simulink model "Optical_Movement_Detection"  (Simulink 7.5)
settings: Solver=ode45  StartTime=0.0  StopTime=inf  RelTol=1e-3
values from neighbouring files (symbols this model uses):
  D = 1    [Copter_Animation.m]
  HSE_Bottom_1 = imresize(imread('D:\GoogleMapsBilder\PAR\HSE_Bottom_1.jpg'), 1)    [TESTS_Optical_Flow_Scenarios.m]
undefined symbols (not defined in the file or in its folder): dfilt, fspecial, imresize, Kanade, Low, Lucas, Rec, SDTV
libraries: simulink x17, dspobslib x12, vipgeotforms x5, dspsigops x4, dspmtrx3 x3, vipanalysis x3, dspstat3 x3, vipconversions x2, dspswit3 x2, vipsrcs x2, dsparch4 x1, dspsrcs4 x1
(part 1 of 2)
settings Model: Creator=roczit00  LastModifiedBy=Anonymos
settings DataIOCC: SaveOutput=off  DSMLogging=off  SaveTime=off
settings DebuggingCC: AlgebraicLoopMsg=none  SolverPrmCheckMsg=none  UnconnectedInputMsg=none  UnconnectedOutputMsg=none  UnconnectedLineMsg=none  StrictBusMsg=Warning

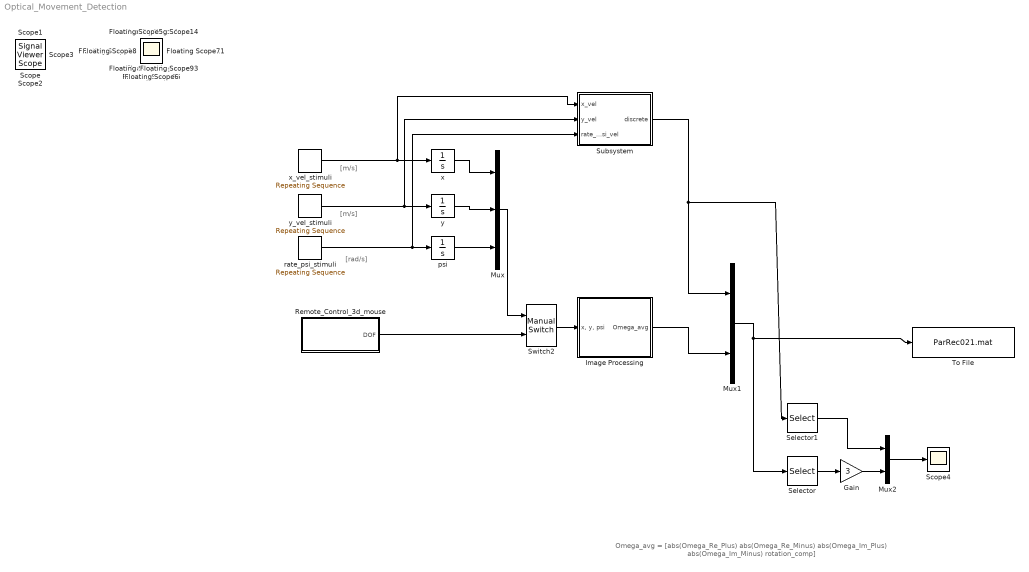
== system Optical_Movement_Detection ==
  note: [m/s]
  note: [m/s]
  note: [rad/s]
  note: Omega_avg = [abs(Omega_Re_Plus) abs(Omega_Re_Minus) abs(Omega_Im_Plus) abs(Omega_Im_Minus) rotation_comp]
  Gain : Gain  Gain=3  ParameterDataType=fixdt(1, 16)  ParameterScaling=2^0  OutDataType=fixdt(1, 16)  OutScaling=2^0
  Image Processing : Subsystem  mask{Ts_Opt=50, Cam_Img_Dim=[300,300], Env_Orig=[1300 1300], Block_Matching_Size=[31,31], Block_Matching_Overlap=[0 0], Block_Matching_Max_Disp=[7 7], Omega_avg_Gain=1/1000, load_cmd=HSE_Bottom_1}
      mask prompts: Ts_Opt "Camera's frames per second (1/SampleTime):"; Cam_Img_Dim "Cameras size of the synthetic image [R C]:"; Env_Orig "Initial image center of environment [R C]:"; Block_Matching_Size "Block size of optical flow block matching algorithm [heigh width]"; Block_Matching_Overlap "Block Overlap [R C] :"; Block_Matching_Max_Disp "Maximum displacement [R C]:"; Omega_avg_Gain "Gain of detected velocity vector"; load_cmd "Load Cmd"
      mask init:
      | set_param(gcb,'MaskSelfModifiable','on')
      mask TabNameString: General,General,General,Block Matching,Block Matching,Block Matching,Block Matching,General
  Mux : Mux  Inputs=3
  Mux1 : Mux  Inputs=2
  Mux2 : Mux  Inputs=2
  Remote_Control_3d_mouse : Subsystem  AncestorBlock=Remote_Control_Library/Remote_Control_3d_mouse
  Scope4 : Scope
      settings: TimeRange=1  YMin=0.25  YMax=4.5  SaveName=ScopeData9
  Selector : Selector  InputPortWidth=8  IndexOptions=Index vector (dialog)  Indices=[4]  OutputSizes=1
  Selector1 : Selector  InputPortWidth=3  IndexOptions=Index vector (dialog)  Indices=[1]  OutputSizes=1
  Subsystem : Subsystem  mask{In_Val_Sample_Time=0.01}
      mask prompts: In_Val_Sample_Time "Sample time"
  Switch2 : simulink/Signal Routing/Manual Switch  SystemSampleTime=-1  sw=1  action=0  varsize=off
  To File : ToFile  Filename=ParRec021.mat  MatrixName=Tfile
  psi : Integrator
  rate_psi_stimuli : simulink/Sources/Repeating Sequence  SystemSampleTime=-1  rep_seq_t=[0,5]  rep_seq_y=[0,-5]
  x : Integrator
  x_vel_stimuli : simulink/Sources/Repeating Sequence  SystemSampleTime=-1  rep_seq_t=[0,10]  rep_seq_y=[0,0]
  y : Integrator
  y_vel_stimuli : simulink/Sources/Repeating Sequence  SystemSampleTime=-1  rep_seq_t=[0,10]  rep_seq_y=[0,0]
  Floating Scope{,1..15} (16 alike) : Scope
      Floating Scope settings: Floating=on  YMin=-40  YMax=90
      Floating Scope1 settings: Floating=on
      Floating Scope10 settings: Floating=on  SaveName=ScopeData12
      Floating Scope11 settings: Floating=on  SaveName=ScopeData13
      Floating Scope12 settings: Floating=on  YMin=-2500  YMax=27500  SaveName=ScopeData14
      Floating Scope13 settings: Floating=on  YMin=3  YMax=7  SaveName=ScopeData15
      Floating Scope14 settings: Floating=on  SaveName=ScopeData16
      Floating Scope15 settings: Floating=on  SaveName=ScopeData17
      Floating Scope2 settings: Floating=on  YMin=-6000  YMax=2500  SaveName=ScopeData2
      Floating Scope3 settings: Floating=on  SaveName=ScopeData3
      Floating Scope4 settings: Floating=on  SaveName=ScopeData4
      Floating Scope5 settings: Floating=on  YMin=-0.7  YMax=0.8  SaveName=ScopeData5
      Floating Scope6 settings: Floating=on  YMin=-1  YMax=1  SaveName=ScopeData6
      Floating Scope7 settings: Floating=on  YMin=-15  YMax=10  SaveName=ScopeData7
      Floating Scope8 settings: Floating=on  YMax=45  SaveName=ScopeData10
      Floating Scope9 settings: Floating=on  YMin=-7  YMax=9  SaveName=ScopeData11
  Scope{,1..3} (4 alike) : SignalViewerScope  IOType=viewer  RefreshTime=0.035000
      Scope settings: YMin=-0.01  YMax=0.1
      Scope2 settings: SaveName=ScopeData2
      Scope3 settings: SaveName=ScopeData3
  wires:
  Remote_Control_3d_mouse/1(DOF) -> Switch2/2
  Mux/1 -> Switch2/1
  Switch2/1 -> Image Processing/1("x, y, psi")
  y_vel_stimuli/1 -> y/1, Subsystem/2(y_vel)
  x_vel_stimuli/1 -> x/1, Subsystem/1(x_vel)
  psi/1 -> Mux/3
  x/1 -> Mux/1
  y/1 -> Mux/2
  Mux1/1 -> Selector/1, To File/1
  Image Processing/1(Omega_avg) -> Mux1/2
  Mux2/1 -> Scope4/1
  Subsystem/1(discrete) -> Mux1/1, Selector1/1
  Selector/1 -> Gain/1
  Gain/1 -> Mux2/2
  Selector1/1 -> Mux2/1
  rate_psi_stimuli/1 -> psi/1, Subsystem/3(rate_psi_vel)

== system Optical_Movement_Detection/Image Processing ==
  note: Image Processing
  "x, y, psi" : Inport
  Allow Optical Flow : dspobslib/DSP Constant  SystemSampleTime=-1  Value=1  SampleMode=Discrete  discreteOutput=Sample-based  continuousOutput=Sample-based  sampTime=inf  framePeriod=2  dataType=boolean  isSigned=on  wordLen=16  udDataType=sfix(16)  fracBitsMode=Best precision  numFracBits=15  InterpretAs1D=-inf  Ts=-inf  FramebasedOutput=-inf
  Disable Optical Flow : dspobslib/DSP Constant  SystemSampleTime=-1  Value=0  SampleMode=Discrete  discreteOutput=Sample-based  continuousOutput=Sample-based  sampTime=inf  framePeriod=2  dataType=boolean  isSigned=on  wordLen=16  udDataType=sfix(16)  fracBitsMode=Best precision  numFracBits=15  InterpretAs1D=-inf  Ts=-inf  FramebasedOutput=-inf
  Input : Subsystem
      mask init:
      | set_param(gcb,'MaskSelfModifiable','on')
  Optical Flow : Subsystem
  Real Video : dspobslib/DSP Constant  SystemSampleTime=-1  Value=0  SampleMode=Discrete  discreteOutput=Sample-based  continuousOutput=Sample-based  sampTime=inf  framePeriod=2  dataType=boolean  isSigned=on  wordLen=16  udDataType=sfix(16)  fracBitsMode=Best precision  numFracBits=15  InterpretAs1D=-inf  Ts=-inf  FramebasedOutput=-inf
  Switch : simulink/Signal Routing/Manual Switch  SystemSampleTime=-1  sw=0  action=0  varsize=off
  Switch1 : simulink/Signal Routing/Manual Switch  SystemSampleTime=-1  sw=1  action=0  varsize=off
  Synthetic Video : dspobslib/DSP Constant  SystemSampleTime=-1  Value=1  SampleMode=Discrete  discreteOutput=Sample-based  continuousOutput=Sample-based  sampTime=inf  framePeriod=2  dataType=boolean  isSigned=on  wordLen=16  udDataType=sfix(16)  fracBitsMode=Best precision  numFracBits=15  InterpretAs1D=-inf  Ts=-inf  FramebasedOutput=-inf
  Omega_avg : Outport
  wires:
  Real Video/1 -> Switch/1
  Synthetic Video/1 -> Switch/2
  Switch/1 -> Input/1(Mode)
  "x, y, psi"/1 -> Input/2("x, y, psi")
  Input/1(Image) -> Optical Flow/1(Image)
  Input/2(I) -> Optical Flow/2(I)
  Allow Optical Flow/1 -> Switch1/1
  Disable Optical Flow/1 -> Switch1/2
  Optical Flow/1(Omega_avg) -> Omega_avg/1
  Switch1/1 -> Optical Flow/Enable

== system Optical_Movement_Detection/Remote_Control_3d_mouse ==
  Demux : Demux  Outputs=3
  Demux1 : Demux  Outputs=3
  Mux2 : Mux  Inputs=3
  Saturation : Saturate  UpperLimit=255  LowerLimit=-255
  Saturation1 : Saturate  UpperLimit=10  LowerLimit=-10
  Saturation2 : Saturate  UpperLimit=10  LowerLimit=-10
  Space Mouse Input : S-Function  AncestorBlock=vrlib/Space Mouse Input  FunctionName=spacemouse  Parameters=Port, OutputType, InitialPosition, InitialRotation, PositionSensitivity, RotationSensitivity, Dominant, NormalizeAngle, DisableTranslation, DisableRotation, PositionLow, PositionUp, EnableLimit  EnableBusSupport=off  mask(Space Mouse Input){Port=USB1, OutputType=Speed, Dominant=off, DisableTranslation=off, DisableRotation=off, NormalizeAngle=off, EnableLimit=on, PositionSensitivity=0.001, RotationSensitivity=0.001, InitialPosition=[0 0 0], InitialRotation=[0 0 0], PositionLow=[0 0 0], PositionUp=[255 255 255]}
      mask prompts: OutputType "Output type:"; Dominant "Dominant mode"; DisableTranslation "Disable position movement"; DisableRotation "Disable rotation movement"; NormalizeAngle "Normalize output angle"; EnableLimit "Limit position"; PositionSensitivity "Position sensitivity:"; RotationSensitivity "Rotation sensitivity:"; InitialPosition "Initial position:"; InitialRotation "Initial rotation:"; PositionLow "Lower position limit:"; PositionUp "Upper position limit:"
      mask help: Space Mouse input device driver.
      mask Help: helpview(fullfile(docroot, 'toolbox', 'sl3d', 'sl3d.map'), 'vr_magellanspacemouse');
      mask StyleString: popup(COM1|COM2|COM3|COM4|USB1|USB2|USB3|USB4|USB),popup(Speed|Position|Viewpoint coordinates),checkbox,checkbox,checkbox,checkbox,checkbox,edit,edit,edit,edit,edit,edit
      mask CallbackString: spacemousemask|spacemousemask|||||spacemousemask||||||
      mask Display:
      | image(imread('spacemouseicon.png'))
      | port_label('output', 1, 'Translation')
      | port_label('output', 2, 'Rotation')
      | port_label('output', 3, 'Buttons')
  x : Integrator
  y : Integrator
  y1 : Integrator
  DOF : Outport
  wires:
  Demux/1 -> Saturation/1  "phi_set"
  Demux/3 -> Saturation1/1  "theta_set"
  Demux1/2 -> Saturation2/1  "psi_set"
  Space Mouse Input/2 -> Demux1/1  "[Kippen, Rollen, Drehen]"
  Space Mouse Input/1 -> Demux/1  "[Trans_X, Trans_Z, Trans_Y]"
  Mux2/1 -> DOF/1
  Saturation1/1 -> y/1
  Saturation2/1 -> y1/1
  Saturation/1 -> x/1
  y1/1 -> Mux2/3
  y/1 -> Mux2/2
  x/1 -> Mux2/1

== system Optical_Movement_Detection/Subsystem ==
  note: discrete [x_vel_d y_vel_d rate_psi_vel_d]
  x_vel : Inport
  y_vel : Inport  Port=2
  rate_psi_vel : Inport  Port=3
  Mux3 : Mux  Inputs=3
  Zero-Order Hold2 : ZeroOrderHold  SampleTime=In_Val_Sample_Time
  Zero-Order Hold3 : ZeroOrderHold  SampleTime=In_Val_Sample_Time
  Zero-Order Hold4 : ZeroOrderHold  SampleTime=In_Val_Sample_Time
  discrete : Outport
  wires:
  Zero-Order Hold2/1 -> Mux3/1
  Zero-Order Hold3/1 -> Mux3/2
  Zero-Order Hold4/1 -> Mux3/3
  x_vel/1 -> Zero-Order Hold2/1
  y_vel/1 -> Zero-Order Hold3/1
  rate_psi_vel/1 -> Zero-Order Hold4/1
  Mux3/1 -> discrete/1

== system Optical_Movement_Detection/Image Processing/Input ==
  Mode : Inport  OutDataType=sfix(16)  OutScaling=2^0
  "x, y, psi" : Inport  Port=2  OutDataType=sfix(16)  OutScaling=2^0
  Color Space  Conversion : vipconversions/Color Space  Conversion  conversion=Obsolete  conversionActive=R'G'B' to intensity  wp_str=D65  rec=Rec. 601 (SDTV)  sys=1125/60/2:1  imagePorts=One multidimensional signal
  Real Video : dspobslib/DSP Constant  SystemSampleTime=-1  Value=0  SampleMode=Discrete  discreteOutput=Sample-based  continuousOutput=Sample-based  sampTime=inf  framePeriod=2  dataType=boolean  isSigned=on  wordLen=16  udDataType=sfix(16)  fracBitsMode=Best precision  numFracBits=15  InterpretAs1D=-inf  Ts=-inf  FramebasedOutput=-inf
  Subsystem : Subsystem
  Synthetic Video Generation : Subsystem  mask(Synthetic Video Generation){dimen=Cam_Img_Dim, origin=Env_Orig, velocity=[100 100], varVelocity=[100 100], varCorner=[100 100], rotation=100, varRotation=100}
      mask prompts: dimen "Size of the synthetic image:"; origin "Initial image center:"; varVelocity "Variance of velocity:"; varCorner "Variance of corner location:"; rotation "Rotation speed (in degrees):"; varRotation "Variation of rotation (in degrees):"
      mask help: Generates a synthetic video.
  Zero-Order Hold1 : ZeroOrderHold  SampleTime=1/Ts_Opt
  Image : Outport
  I : Outport  Port=2
  wires:
  Mode/1 -> Synthetic Video Generation/Enable
  Color Space  Conversion/1 -> I/1
  Real Video/1 -> Subsystem/Enable
  Synthetic Video Generation/1(Image) -> Color Space  Conversion/1, Image/1
  "x, y, psi"/1 -> Zero-Order Hold1/1
  Zero-Order Hold1/1 -> Synthetic Video Generation/1("x, y, psi")

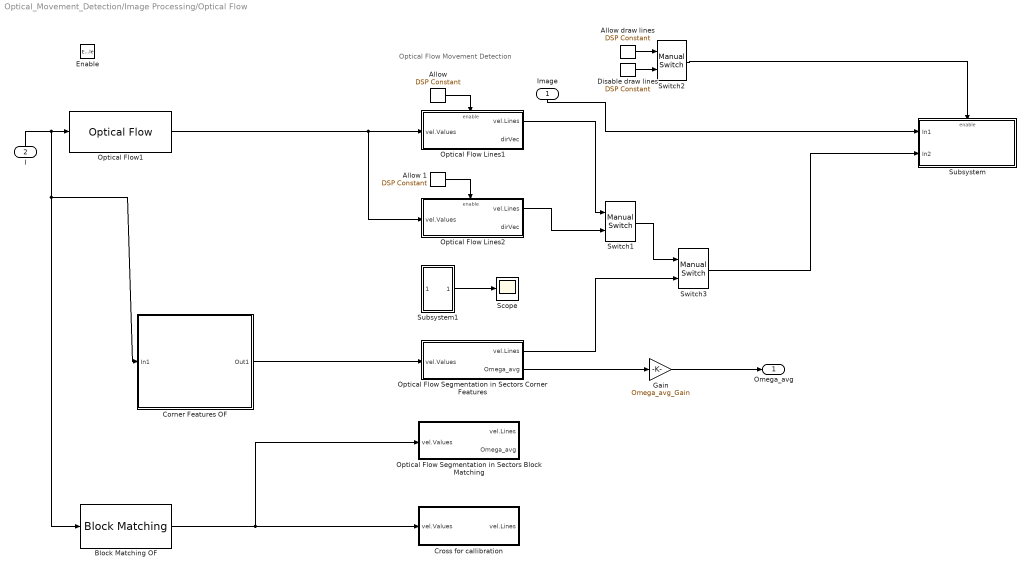
== system Optical_Movement_Detection/Image Processing/Optical Flow ==
  note: Optical Flow Movement Detection
  Image : Inport
  I : Inport  Port=2
  Enable : EnablePort  PropagateVarSize=During execution
  "Allow " : dspobslib/DSP Constant  SystemSampleTime=-1  Value=0  SampleMode=Discrete  discreteOutput=Sample-based  continuousOutput=Sample-based  sampTime=inf  framePeriod=2  dataType=boolean  isSigned=on  wordLen=16  udDataType=sfix(16)  fracBitsMode=Best precision  numFracBits=15  InterpretAs1D=-inf  Ts=-inf  FramebasedOutput=-inf
  Allow 1 : dspobslib/DSP Constant  SystemSampleTime=-1  Value=0  SampleMode=Discrete  discreteOutput=Sample-based  continuousOutput=Sample-based  sampTime=inf  framePeriod=2  dataType=boolean  isSigned=on  wordLen=16  udDataType=sfix(16)  fracBitsMode=Best precision  numFracBits=15  InterpretAs1D=-inf  Ts=-inf  FramebasedOutput=-inf
  Allow draw lines : dspobslib/DSP Constant  SystemSampleTime=-1  Value=1  SampleMode=Discrete  discreteOutput=Sample-based  continuousOutput=Sample-based  sampTime=inf  framePeriod=2  dataType=boolean  isSigned=on  wordLen=16  udDataType=sfix(16)  fracBitsMode=Best precision  numFracBits=15  InterpretAs1D=-inf  Ts=-inf  FramebasedOutput=-inf
  Block Matching OF : vipanalysis/Block Matching  DialogController=vipDDGCreate  DialogControllerArgs=DataTag8  SystemSampleTime=-1  which2img=Current frame and N-th frame back  N=1  searchMethod=Exhaustive  blockSize=Block_Matching_Size  overlapping=Block_Matching_Overlap  maxDisplacement=Block_Matching_Max_Disp  matchCriteria=Mean absolute difference (MAD)  outVelForm=Horizontal and vertical components in complex form  outputMode=Binary point scaling  outputWordLength=32  outputFracLength=0  accumMode=Binary point scaling  accumWordLength=64  accumFracLength=0  prodOutputMode=Binary point scaling  prodOutputWordLength=32  prodOutputFracLength=0  roundingMode=Ceiling  overflowMode=off
      link override Delay: dly_unit=Frames  delay=N
  Corner Features OF : Subsystem
  Cross for callibration : Subsystem  mask(Optical Flow Lines){scaleFactor=10}
      mask prompts: scaleFactor "Motion vector gain:"
      mask help: Generates the coordinate points of optical flow lines.
      mask Help: Generates the coordinate points of optical flow lines. Look under its mask to see the implementation details.
  Disable draw lines : dspobslib/DSP Constant  SystemSampleTime=-1  Value=0  SampleMode=Discrete  discreteOutput=Sample-based  continuousOutput=Sample-based  sampTime=inf  framePeriod=2  dataType=boolean  isSigned=on  wordLen=16  udDataType=sfix(16)  fracBitsMode=Best precision  numFracBits=15  InterpretAs1D=-inf  Ts=-inf  FramebasedOutput=-inf
  Gain : Gain  Gain=Omega_avg_Gain  ParameterDataType=fixdt(1, 16)  ParameterScaling=2^0  OutDataType=fixdt(1, 16)  OutScaling=2^0
  Optical Flow Lines1 : Subsystem  mask(Optical Flow Lines){scaleFactor=0.0008}
      mask prompts: scaleFactor "Motion vector gain:"
      mask help: Generates the coordinate points of optical flow lines.
      mask Help: Generates the coordinate points of optical flow lines. Look under its mask to see the implementation details.
  Optical Flow Lines2 : Subsystem  mask(Optical Flow Lines){scaleFactor=5}
      mask prompts: scaleFactor "Motion vector gain:"
      mask help: Generates the coordinate points of optical flow lines.
      mask Help: Generates the coordinate points of optical flow lines. Look under its mask to see the implementation details.
  Optical Flow Segmentation in Sectors Block Matching : Subsystem  mask(Optical Flow Lines){scaleFactor=10}
      mask prompts: scaleFactor "Motion vector gain:"
      mask help: Generates the coordinate points of optical flow lines.
      mask Help: Generates the coordinate points of optical flow lines. Look under its mask to see the implementation details.
  Optical Flow Segmentation in Sectors Corner Features : Subsystem  mask(Optical Flow Lines){scaleFactor=10}
      mask prompts: scaleFactor "Motion vector gain:"
      mask help: Generates the coordinate points of optical flow lines.
      mask Help: Generates the coordinate points of optical flow lines. Look under its mask to see the implementation details.
  Optical Flow1 : vipanalysis/Optical Flow  DialogController=vipDDGCreate  DialogControllerArgs=DataTag13  SystemSampleTime=-1  method=Lucas-Kanade  gradMethod=Derivative of Gaussian  which2img=Current frame and N-th frame back  N=1  outVelForm=Horizontal and vertical components in complex form  lambda=1  stop_criteria=When maximum number of iterations is reached  maxAllowAbsDiff=eps  maxIter=10  numInports=3  sigmaS=1.5  sigmaW=1  eigTh=0.0039  discardNormalFlow=on  outputCurrentImage=off  prodOutputMode=Binary point scaling  prodOutputWordLength=32  prodOutputFracLength=20  outputMode=Binary point scaling  outputWordLength=32  outputFracLength=20  roundingMode=Nearest  overflowMode=on
  Scope : Scope
      settings: YMin=0  YMax=10  SaveName=ScopeData8
  Subsystem : Subsystem
  Subsystem1 : Subsystem
  Switch1 : simulink/Signal Routing/Manual Switch  SystemSampleTime=-1  sw=0  action=0  varsize=off
  Switch2 : simulink/Signal Routing/Manual Switch  SystemSampleTime=-1  sw=1  action=0  varsize=off
  Switch3 : simulink/Signal Routing/Manual Switch  SystemSampleTime=-1  sw=0  action=0  varsize=on
  Omega_avg : Outport
  wires:
  Image/1 -> Subsystem/1(In1)
  I/1 -> Optical Flow1/1, Corner Features OF/1(In1), Block Matching OF/1
  Allow draw lines/1 -> Switch2/1
  Disable draw lines/1 -> Switch2/2
  Switch2/1 -> Subsystem/Enable
  Subsystem1/1(angle) -> Scope/1
  Optical Flow Lines2/1(vel.Lines) -> Switch1/2
  Optical Flow Lines1/1(vel.Lines) -> Switch1/1
  Optical Flow1/1 -> Optical Flow Lines1/1(vel.Values), Optical Flow Lines2/1(vel.Values)
  Optical Flow Segmentation in Sectors Corner Features/1(vel.Lines) -> Switch3/2
  Switch1/1 -> Switch3/1
  "Allow "/1 -> Optical Flow Lines1/Enable
  Allow 1/1 -> Optical Flow Lines2/Enable
  Optical Flow Segmentation in Sectors Corner Features/2(Omega_avg) -> Gain/1
  Block Matching OF/1 -> Cross for callibration/1(vel.Values), Optical Flow Segmentation in Sectors Block Matching/1(vel.Values)
  Switch3/1 -> Subsystem/2(In2)
  Gain/1 -> Omega_avg/1
  Corner Features OF/1(Out1) -> Optical Flow Segmentation in Sectors Corner Features/1(vel.Values)

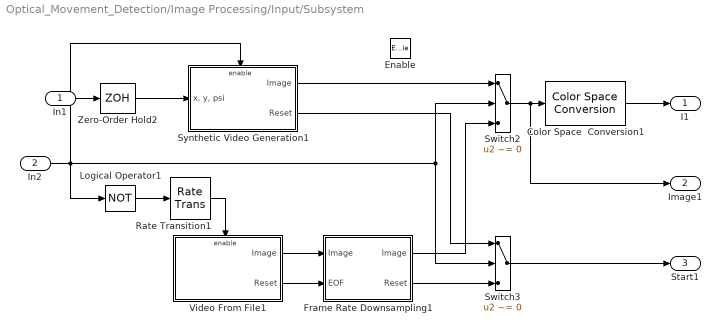
== system Optical_Movement_Detection/Image Processing/Input/Subsystem ==
  In1 : Inport
  In2 : Inport  Port=2
  Enable : EnablePort  PropagateVarSize=During execution
  Color Space  Conversion1 : vipconversions/Color Space  Conversion  conversion=Obsolete  conversionActive=R'G'B' to intensity  wp_str=D65  rec=Rec. 601 (SDTV)  sys=1125/60/2:1  imagePorts=One multidimensional signal
  Frame Rate Downsampling1 : Subsystem  mask(Select Video Frames){frameRate=1}
      mask prompts: frameRate "N:"
      mask help: Downsample the video sequence by processing every Nth frame.
      mask init:
      | switch frameRate
      |     case 1,
      |         icon = sprintf('Select\nAll Frames');
      |     case 2,
      |         icon = sprintf('Select Every\n2nd Frame');
      |     case 3,
      |         icon = sprintf('Select Every\n3rd Frame');
      |     otherwise,
      |         icon = sprintf('Select Every\n%dth Frame',frameRate);
      | end
      mask Display: disp(icon);
  Logical Operator1 : Logic  Operator=NOT  AllPortsSameDT=off  OutDataTypeMode=boolean  OutDataTypeStr=boolean
  Rate Transition1 : RateTransition  OutPortSampleTimeOpt=Inherit
  Switch2 : Switch  Criteria=u2 ~= 0  OutDataType=sfix(16)  OutScaling=2^0
  Switch3 : Switch  Criteria=u2 ~= 0  OutDataType=sfix(16)  OutScaling=2^0
  Synthetic Video Generation1 : Subsystem  mask(Synthetic Video Generation){dimen=[288 352], origin=[509 765], velocity=[5 10], varVelocity=[8 5], varCorner=[10 10], rotation=1, varRotation=0.2}
      mask prompts: dimen "Size of the synthetic image:"; origin "Initial image center:"; varVelocity "Variance of velocity:"; varCorner "Variance of corner location:"; rotation "Rotation speed (in degrees):"; varRotation "Variation of rotation (in degrees):"
      mask help: Generates a synthetic video.
  Video From File1 : Subsystem
  Zero-Order Hold2 : ZeroOrderHold  SampleTime=0.01
  I1 : Outport
  Image1 : Outport  Port=2
  Start1 : Outport  Port=3
  wires:
  Switch3/1 -> Start1/1
  Switch2/1 -> Image1/1, Color Space  Conversion1/1
  Logical Operator1/1 -> Rate Transition1/1
  Rate Transition1/1 -> Video From File1/Enable
  Synthetic Video Generation1/2(Reset) -> Switch3/1
  Synthetic Video Generation1/1(Image) -> Switch2/1
  In2/1 -> Logical Operator1/1, Switch3/2, Switch2/2, Synthetic Video Generation1/Enable
  Video From File1/1(Image) -> Frame Rate Downsampling1/1(Image)
  Video From File1/2(Reset) -> Frame Rate Downsampling1/2(EOF)
  Frame Rate Downsampling1/1("Image ") -> Switch2/3
  Frame Rate Downsampling1/2(Reset) -> Switch3/3
  Zero-Order Hold2/1 -> Synthetic Video Generation1/1("x, y, psi")
  Color Space  Conversion1/1 -> I1/1
  In1/1 -> Zero-Order Hold2/1

== system Optical_Movement_Detection/Image Processing/Input/Synthetic Video Generation ==
  "x, y, psi" : Inport  OutDataType=sfix(16)  OutScaling=2^0
  Enable : EnablePort  PropagateVarSize=During execution
  N-Sample Enable : dspswit3/N-Sample Enable  N=1  ActiveLevel=Low (0)  reset=off  TriggerType=Rising edge  Ts=-1  DataType=Logical
  Read Image : Subsystem
      settings: AttributesFormatString=Load image only at the beginning of simulation
  Synthesize Video : Subsystem  mask{dimen=dimen, origin=origin, velocity=velocity, varVelocity=varVelocity, varCorner=varCorner, rotation=rotation, varRotation=varRotation}
      mask prompts: dimen "Size of the synthetic image:"; origin "Initial image center:"; varVelocity "Variance of velocity:"; varCorner "Variance of corner location:"; rotation "Rotation speed:"; varRotation "Variation of rotation:"
  Image : Outport
  Reset : Outport  Port=2  InitialOutput=1
  wires:
  Read Image/2(Size) -> Synthesize Video/2(Size)
  Read Image/1(Image) -> Synthesize Video/1("Image ")
  N-Sample Enable/1 -> Read Image/Enable
  Synthesize Video/2(Reset) -> Reset/1
  Synthesize Video/1(Image) -> Image/1
  "x, y, psi"/1 -> Synthesize Video/3("x, y, psi")

== system Optical_Movement_Detection/Image Processing/Optical Flow/Corner Features OF ==
  In1 : Inport
  Compare : RelationalOperator  LogicOutDataTypeMode=boolean  OutDataTypeStr=boolean  ZeroCross=off  InputSameDT=on
  Corner Detection : vipanalysis/Corner Detection  DialogController=vipDDGCreate  DialogControllerArgs=DataTag9  SystemSampleTime=-1  method=Minimum eigenvalue (Shi & Tomasi)  factor=0.04  filter=fspecial('gaussian', [1 5], 1.5)  thrInten=0.1  thrAngle=157.5  output=Corner location  outputInUse=Corner location  maxNum=75  thrMetric=0.001  neighborSize=[21 21]  isOutVarDim=on  accumMode=Binary point scaling  accumWordLength=32  accumFracLength=0  prodOutputMode=Binary point scaling  prodOutputWordLength=32  prodOutputFracLength=0  memoryMode=Binary point scaling  memoryWordLength=32  memoryFracLength=0  firstCoeffMode=Specify word length  firstCoeffWordLength=16  firstCoeffFracLength=16  roundingMode=Floor  overflowMode=off
  Corner Matching : Subsystem  mask(Corner Matching){winLen=9, maxNum=75, threshold=81}
      mask prompts: winLen "Block size used in corner matching:"; maxNum "Maximum number of points:"; threshold "Maximum feature difference for matching points:"
      mask help: Find out matching corners in the current and previous video frames.
  Embedded MATLAB Function : Stateflow chart  TreatAsAtomicUnit=on
  Estimate Geometric Transformation : vipgeotforms/Estimate Geometric Transformation  DialogController=vipDDGCreate  DialogControllerArgs=DataTag12  tformType=Projective  isRandomSampling=on  algMethod=Random Sample Consensus (RANSAC)  numMethod=Desired confidence  isStopSampling=on  percentStop=75  distanceAlg=1  distanceGeo=1.5  sampleNum=500  maxSampleNum=500  desiredConfidence=99  isRefineTForm=on  isOutputInlier=on  outDT4IntInput=Obsolete10a  outDT4IntInputActive=Double  isVarSizeAllowed=off  isReleaseMode=on
  Number of  Inliers Threshold : Constant  OutDataType=sfix(16)  OutScaling=1  OutDataTypeStr=Inherit: Inherit via back propagation  SampleTime=-1
  Scope : Scope
      settings: YMax=1  SaveName=ScopeData18
  Sum of Elements : Sum  Inputs=+  OutDataType=sfix(16)  OutScaling=2^-10
  fps : Constant  Value=1/Ts_Opt  OutDataType=sfix(16)  OutScaling=1  OutDataTypeStr=Inherit: Inherit via back propagation  SampleTime=-1
  Out1 : Outport
  wires:
  Corner Matching/1(Pts1) -> Estimate Geometric Transformation/1
  Corner Matching/2(Pts2) -> Estimate Geometric Transformation/2
  Corner Matching/3("Num ") -> Estimate Geometric Transformation/3
  Corner Detection/1 -> Corner Matching/2(Pts)
  Corner Detection/2 -> Corner Matching/3(Num)
  Estimate Geometric Transformation/1 -> Embedded MATLAB Function/1(Tform)
  In1/1 -> Corner Matching/1(I), Corner Detection/1
  Embedded MATLAB Function/1(vec) -> Out1/1
  Compare/1 -> Embedded MATLAB Function/2(allowNewCalc)
  Number of  Inliers Threshold/1 -> Compare/2
  Sum of Elements/1 -> Compare/1
  Estimate Geometric Transformation/2 -> Sum of Elements/1
  Embedded MATLAB Function/2(rot) -> Scope/1
  fps/1 -> Embedded MATLAB Function/3(TsOpt)

== system Optical_Movement_Detection/Image Processing/Optical Flow/Cross for callibration ==
  vel.Values : Inport  OutDataType=sfix(16)  OutScaling=2^0
  " " : dspobslib/DSP Constant  SystemSampleTime=-1  Value=Cam_Img_Dim  SampleMode=Discrete  discreteOutput=Sample-based  continuousOutput=Sample-based  sampTime=inf  framePeriod=2  dataType=double  isSigned=on  wordLen=16  udDataType=sfix(16)  fracBitsMode=Best precision  numFracBits=15  InterpretAs1D=-inf  Ts=-inf  FramebasedOutput=-inf
  Optical Flow Lines1 : Stateflow chart  TreatAsAtomicUnit=on
  vel.Lines : Outport  OutDataType=sfix(16)  OutScaling=2^0
  wires:
  Optical Flow Lines1/1(vel_Lines) -> vel.Lines/1
  vel.Values/1 -> Optical Flow Lines1/1(vel_Values)
  " "/1 -> Optical Flow Lines1/2(Cam_Img_Dim)

== system Optical_Movement_Detection/Image Processing/Optical Flow/Optical Flow Lines1 ==
  vel.Values : Inport  OutDataType=sfix(16)  OutScaling=2^0
  Enable : EnablePort  PropagateVarSize=During execution
  Optical Flow Lines1 : Stateflow chart  TreatAsAtomicUnit=on
  vel.Lines : Outport  OutDataType=sfix(16)  OutScaling=2^0
  dirVec : Outport  Port=2  OutDataType=sfix(16)  OutScaling=2^0
  wires:
  Optical Flow Lines1/1(vel_Lines) -> vel.Lines/1
  vel.Values/1 -> Optical Flow Lines1/1(vel_Values)
  Optical Flow Lines1/2(dir_Vec) -> dirVec/1

== system Optical_Movement_Detection/Image Processing/Optical Flow/Optical Flow Lines2 ==
  vel.Values : Inport  OutDataType=sfix(16)  OutScaling=2^0
  Enable : EnablePort  PropagateVarSize=During execution
  Optical Flow Lines1 : Stateflow chart  TreatAsAtomicUnit=on
  vel.Lines : Outport  OutDataType=sfix(16)  OutScaling=2^0
  dirVec : Outport  Port=2  OutDataType=sfix(16)  OutScaling=2^0
  wires:
  Optical Flow Lines1/1(vel_Lines) -> vel.Lines/1
  vel.Values/1 -> Optical Flow Lines1/1(vel_Values)
  Optical Flow Lines1/2(dir_Vec) -> dirVec/1

== system Optical_Movement_Detection/Image Processing/Optical Flow/Optical Flow Segmentation in Sectors Block Matching ==
  note: Omega_avg = [abs(Omega_Re_Plus) abs(Omega_Re_Minus) abs(Omega_Im_Plus) abs(Omega_Im_Minus) rotation_comp]
  vel.Values : Inport  OutDataType=sfix(16)  OutScaling=2^0
  " " : dspobslib/DSP Constant  SystemSampleTime=-1  Value=Cam_Img_Dim  SampleMode=Discrete  discreteOutput=Sample-based  continuousOutput=Sample-based  sampTime=inf  framePeriod=2  dataType=double  isSigned=on  wordLen=16  udDataType=sfix(16)  fracBitsMode=Best precision  numFracBits=15  InterpretAs1D=-inf  Ts=-inf  FramebasedOutput=-inf
  Optical Flow Lines1 : Stateflow chart  TreatAsAtomicUnit=on
  vel.Lines : Outport  OutDataType=sfix(16)  OutScaling=2^0
  Omega_avg : Outport  Port=2  OutDataType=sfix(16)  OutScaling=2^0
  wires:
  Optical Flow Lines1/1(vel_Lines) -> vel.Lines/1
  vel.Values/1 -> Optical Flow Lines1/1(vel_Values)
  Optical Flow Lines1/2(Omega_avg) -> Omega_avg/1
  " "/1 -> Optical Flow Lines1/2(Cam_Img_Dim)

== system Optical_Movement_Detection/Image Processing/Optical Flow/Optical Flow Segmentation in Sectors Corner Features ==
  note: Omega_avg = [abs(Omega_Re_Plus) abs(Omega_Re_Minus) abs(Omega_Im_Plus) abs(Omega_Im_Minus) rotation_comp]
  vel.Values : Inport  OutDataType=sfix(16)  OutScaling=2^0
  " " : dspobslib/DSP Constant  SystemSampleTime=-1  Value=Cam_Img_Dim  SampleMode=Discrete  discreteOutput=Sample-based  continuousOutput=Sample-based  sampTime=inf  framePeriod=2  dataType=double  isSigned=on  wordLen=16  udDataType=sfix(16)  fracBitsMode=Best precision  numFracBits=15  InterpretAs1D=-inf  Ts=-inf  FramebasedOutput=-inf
  Optical Flow Lines1 : Stateflow chart  TreatAsAtomicUnit=on
  vel.Lines : Outport  OutDataType=sfix(16)  OutScaling=2^0
  Omega_avg : Outport  Port=2  OutDataType=sfix(16)  OutScaling=2^0
  wires:
  Optical Flow Lines1/1(vel_Lines) -> vel.Lines/1
  vel.Values/1 -> Optical Flow Lines1/1(vel_Values)
  Optical Flow Lines1/2(Omega_avg) -> Omega_avg/1
  " "/1 -> Optical Flow Lines1/2(Cam_Img_Dim)

== system Optical_Movement_Detection/Image Processing/Optical Flow/Subsystem ==
  In1 : Inport
  In2 : Inport  Port=2
  Enable : EnablePort  PropagateVarSize=During execution
  Draw Shapes1 : viptextngfix/Draw Shapes  DialogController=vipDDGCreate  DialogControllerArgs=DataTag14  shape=Lines  fill=off  fillClrSource=Specify via dialog  display=User-specified value  intensity=200  color=[255 255 0]  opacity=0.6  viewport=Entire image  antialiasing=off  inType=Obsolete  imagePorts=One multidimensional signal  prodOutputMode=Binary point scaling  prodOutputWordLength=32  prodOutputFracLength=14  memoryMode=Specify word length  memoryWordLength=16  memoryFracLength=15  roundingMode=Floor  overflowMode=off
  To Video Display : vipsnks/To Video Display  DialogControllerArgs=DataTag15  inputType=Obsolete  imagePorts=One multidimensional signal  OutputDevice=On-screen video monitor  fullScreen=off  videoWindowX=527  videoWindowY=141  saveWindowSize=off  videoWindowWidth=300  videoWindowHeight=300  dataOrg=Column-major  openAtMdlStart=on  isWindowOpen=on
  wires:
  Draw Shapes1/1 -> To Video Display/1
  In1/1 -> Draw Shapes1/1
  In2/1 -> Draw Shapes1/2

== system Optical_Movement_Detection/Image Processing/Optical Flow/Subsystem1 ==
  In1 : Inport
  Complex to Magnitude-Angle : ComplexToMagnitudeAngle
  Demux : Demux  Outputs=2
  Gain : Gain  ParameterDataType=fixdt(1, 16)  ParameterScaling=2^0  OutDataType=fixdt(1, 16)  OutScaling=2^0
  Maximum : dspstat3/Maximum  DialogController=dspDDGCreate  DialogControllerArgs=DataTag16  fcn=Value and Index  reset=None  indexBase=One  operateOver=Entire input  Dimension=1  colComp=off  operation=maximum  roiEnable=off  roiType=Lines  roiPortion=Entire ROI  roiOutput=Individual statistics for each ROI  roiFlag=off  accumDataTypeStr=Inherit: Same as product output  accumLastDataTypeStr=Inherit: Same as product output  roundingMode=Floor  overflowMode=on
  Median : dspstat3/Median  DialogController=dspDDGCreate  DialogControllerArgs=DataTag17  sortAlg=Quick sort  directionMode=Entire input  dimension=2  treatSBRowAsCol=on  outputMin=[]  outputMax=[]  accumDataTypeStr=Inherit: Same as product output  accumLastDataTypeStr=Inherit: Same as product output  roundingMode=Ceiling  overflowMode=on
      settings: allowOverrides=off
  Product : Product  OutDataType=fixdt(1, 16)  OutScaling=2^0  RndMeth=Zero
  Selector : Selector  NumberOfDimensions=2  InputPortWidth=3  IndexOptions=Index vector (port),Index vector (port)  Indices=[0],1  OutputSizes=1,1
  Switch2 : simulink/Signal Routing/Manual Switch  SystemSampleTime=-1  sw=0  action=0  varsize=off
  angle : Outport  OutDataType=fixdt(1, 16)  OutScaling=2^0
  wires:
  In1/1 -> Complex to Magnitude-Angle/1
  Complex to Magnitude-Angle/1 -> Maximum/1, Median/1
  Complex to Magnitude-Angle/2 -> Selector/1
  Demux/1 -> Selector/2
  Gain/1 -> angle/1
  Demux/2 -> Selector/3
  Maximum/1 -> Product/1
  Selector/1 -> Product/2
  Maximum/2 -> Demux/1
  Product/1 -> Switch2/1
  Median/1 -> Switch2/2
  Switch2/1 -> Gain/1

== system Optical_Movement_Detection/Image Processing/Input/Subsystem/Frame Rate Downsampling1 ==
  Image : Inport  OutDataType=sfix(16)  OutScaling=2^0
  EOF : Inport  Port=2  OutDataType=sfix(16)  OutScaling=2^0
  Compare To Zero : simulink/Logic and Bit Operations/Compare To Zero  SystemSampleTime=-1  relop=>  LogicOutDataTypeMode=boolean  ZeroCross=off
  Data Type Conversion : DataTypeConversion  OutDataTypeMode=single  OutDataType=sfix(16)  OutScaling=2^0  OutDataTypeStr=single
  Digital Filter : dsparch4/Digital Filter  DialogController=dspdialog.DigitalFilter  DialogControllerArgs=DataTag0  TypePopup=FIR (all zeros)  IIRFiltStruct=Direct form II transposed  AllPoleFiltStruct=Direct form  FIRFiltStruct=Direct form  CoeffSource=Specify via dialog  NumCoeffs=ones(1, frameRate)  DenCoeffs=[1 0.1]  BiQuadCoeffs=[1 0.3 0.4 1 0.1 0.2]  LatticeCoeffs=[0.2 0.4]  denIgnore=on  FiltPerSampPopup=One filter per frame  IC=0  ICnum=0  ICden=0  roundingMode=Floor  overflowMode=off  ScaleValues=1  scaleValueFracLength=14  stageInFracLength=15  stageOutFracLength=15  FilterSource=Specify via dialog  dfiltObjectName=dfilt.dffir([1 2 1])
  Downsample : dspsigops/Downsample  N=frameRate  phase=0  ic=0  smode=Allow multirate  fmode=Maintain input frame size
  Downsample3 : dspsigops/Downsample  N=frameRate  phase=0  ic=0  smode=Allow multirate  fmode=Maintain input frame size
  Unit Delay : UnitDelay  X0=1  SampleTime=-1
  "Image " : Outport  OutDataType=sfix(16)  OutScaling=2^0
  Reset : Outport  Port=2
  wires:
  Digital Filter/1 -> Compare To Zero/1
  Data Type Conversion/1 -> Digital Filter/1
  Compare To Zero/1 -> Unit Delay/1
  Downsample3/1 -> Reset/1
  EOF/1 -> Data Type Conversion/1
  Unit Delay/1 -> Downsample3/1
  Image/1 -> Downsample/1
  Downsample/1 -> "Image "/1

== system Optical_Movement_Detection/Image Processing/Input/Subsystem/Synthetic Video Generation1 ==
  "x, y, psi" : Inport  OutDataType=sfix(16)  OutScaling=2^0
  Enable : EnablePort  PropagateVarSize=During execution
  N-Sample Enable : dspswit3/N-Sample Enable  N=1  ActiveLevel=Low (0)  reset=off  TriggerType=Rising edge  Ts=-1  DataType=Logical
  Read Image : Subsystem
      settings: AttributesFormatString=Load image only at the beginning of simulation
  Synthesize Video : Subsystem  mask{dimen=dimen, origin=origin, velocity=velocity, varVelocity=varVelocity, varCorner=varCorner, rotation=rotation, varRotation=varRotation}
      mask prompts: dimen "Size of the synthetic image:"; origin "Initial image center:"; varVelocity "Variance of velocity:"; varCorner "Variance of corner location:"; rotation "Rotation speed:"; varRotation "Variation of rotation:"
  Image : Outport
  Reset : Outport  Port=2  InitialOutput=1
  wires:
  Read Image/2(Size) -> Synthesize Video/2(Size)
  Read Image/1(Image) -> Synthesize Video/1("Image ")
  N-Sample Enable/1 -> Read Image/Enable
  Synthesize Video/2(Reset) -> Reset/1
  Synthesize Video/1(Image) -> Image/1
  "x, y, psi"/1 -> Synthesize Video/3("x, y, psi")

== system Optical_Movement_Detection/Image Processing/Input/Subsystem/Video From File1 ==
  Enable : EnablePort  PropagateVarSize=During execution
  From Multimedia File : dspsrcs4/From Multimedia File  DialogController=dspDDGCreate  DialogControllerArgs=DataTag4  inputFilename=D:\_HSE\_ARBEIT\eclipse-cpp-galileo-SR1-win32\Workspace2\MASTER_THESIS_PRJ\scratch\Ground_Videos\grey_amorphic_flow_tiles_variable_light.avi  loop=on  numPlays=inf  outputStreams=Video only  videoDataType=single  audioDataType=int16  inheritSampleTime=on  userDefinedSampleTime=1/30  noAudioOutput=off  isIntensityVideo=off  fourcc=RGB  colorVideoFormat=One multidimensional signal  outputEOF=on  dataOrg=Column-major  audioFrameSize=1024  computeAudioFrameSize=off
  Image : Outport
  Reset : Outport  Port=2
  wires:
  From Multimedia File/1 -> Image/1
  From Multimedia File/2 -> Reset/1

== system Optical_Movement_Detection/Image Processing/Input/Synthetic Video Generation/Read Image ==
  Enable : EnablePort  PropagateVarSize=During execution
  Image From Workspace : vipsrcs/Image From Workspace  Tag=vipblks_nd  SystemSampleTime=-1  ImageValue=load_cmd  Ts=inf  imagePorts=One multidimensional signal  ImageDataType=single  Signed=on  WordLength=16  sdImageDataType=sfix(16)  FractionLengthMode=User-defined  FractionLength=15  OutPortLabels=R|G|B
  Probe : Probe  ProbeWidth=off  ProbeSampleTime=off  ProbeComplexSignal=off  ProbeSignalDimensions=on  ProbeDimensionsDataType=single
  Image : Outport  InitialOutput=0
  Size : Outport  Port=2
  wires:
  Image From Workspace/1 -> Probe/1, Image/1
  Probe/1 -> Size/1

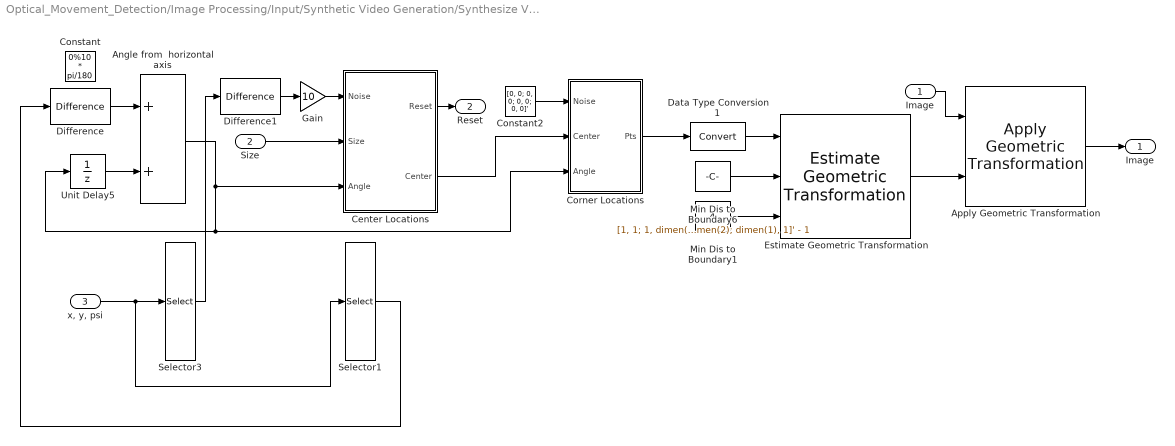
== system Optical_Movement_Detection/Image Processing/Input/Synthetic Video Generation/Synthesize Video ==
  "Image " : Inport  OutDataType=sfix(16)  OutScaling=2^0
  Size : Inport  Port=2  OutDataType=sfix(16)  OutScaling=2^0
  "x, y, psi" : Inport  Port=3  OutDataType=sfix(16)  OutScaling=2^0
  Angle from  horizontal axis : Sum  OutDataType=sfix(16)  OutScaling=2^-10
  Apply Geometric Transformation : vipgeotforms/Apply Geometric Transformation  DialogController=vipDDGCreate  DialogControllerArgs=DataTag5  tformSource=Input port  tformValue=[1 0 0; 0 1 0; 0 0 1]  approxProjectiveFlag=off  errorTolerance=1.0  roiMethod=Whole input image  roiSource=Specify via dialog  roiBBox=[0 0 128 256]  roiVertice=[0 0 10 12 20 22]  inputClipFlag=off  interpolationMethod=Bilinear  fillValue=0  viewPortMethod=Specify via dialog  outputSize=dimen  outputLoc=[0 0]  outputClipFlag=off
  Center Locations : Subsystem
  Constant : Constant  Value=0%10 * pi/180  OutDataType=fixdt(1, 16)  OutScaling=2^0
  Constant2 : Constant  Value=[0, 0; 0, 0; 0, 0; 0, 0]'  OutDataType=fixdt(1, 16)  OutScaling=2^0
  Corner Locations : Subsystem
  Data Type Conversion1 : DataTypeConversion  OutDataType=sfix(16)  OutScaling=2^0
  Difference : simulink/Discrete/Difference  SystemSampleTime=-1  ICPrevInput=0.0  OutMin=[]  OutMax=[]  OutDataType=fixdt(1, 16)  OutScaling=2^-10  DoSatur=off
  Difference1 : simulink/Discrete/Difference  SystemSampleTime=-1  ICPrevInput=0.0  OutMin=[]  OutMax=[]  OutDataType=fixdt(1, 16)  OutScaling=2^-10  DoSatur=off
  Estimate Geometric Transformation : vipgeotforms/Estimate Geometric Transformation  DialogController=vipDDGCreate  DialogControllerArgs=DataTag7  tformType=Projective  isRandomSampling=off  algMethod=Random Sample Consensus (RANSAC)  numMethod=Specified value  isStopSampling=off  percentStop=75  distanceAlg=1.5  distanceGeo=1.5  sampleNum=100  maxSampleNum=200  desiredConfidence=99  isRefineTForm=off  isOutputInlier=off  outDT4IntInput=Obsolete10a  outDT4IntInputActive=Single  isVarSizeAllowed=off  isReleaseMode=on
  Gain : Gain  Gain=10  ParameterDataType=fixdt(1, 16)  ParameterScaling=2^0  OutDataType=fixdt(1, 16)  OutScaling=2^0
  Min Dis to Boundary1 : Constant  Value=4  OutDataType=sfix(16)  OutScaling=2^0  OutDataTypeStr=Inherit: Inherit via back propagation
  Min Dis to Boundary6 : Constant  Value=[1, 1; 1, dimen(2); dimen(1), dimen(2); dimen(1), 1]' - 1  OutDataType=sfix(16)  OutScaling=2^0  OutDataTypeStr=Inherit: Inherit via back propagation
  Selector1 : Selector  InputPortWidth=3  IndexOptions=Index vector (dialog)  Indices=[3]  OutputSizes=1
  Selector3 : Selector  InputPortWidth=3  IndexOptions=Index vector (dialog)  Indices=[2 1]  OutputSizes=1
  Unit Delay5 : UnitDelay  X0=-pi/12  SampleTime=-1
  Image : Outport  OutDataType=sfix(16)  OutScaling=2^0
  Reset : Outport  Port=2  OutDataType=sfix(16)  OutScaling=2^0
  wires:
  Constant2/1 -> Corner Locations/1(Noise)
  Angle from  horizontal axis/1 -> Center Locations/3(Angle), Corner Locations/3(Angle), Unit Delay5/1
  Center Locations/1(Reset) -> Reset/1
  Size/1 -> Center Locations/2(Size)
  Min Dis to Boundary6/1 -> Estimate Geometric Transformation/2
  Min Dis to Boundary1/1 -> Estimate Geometric Transformation/3
  Data Type Conversion1/1 -> Estimate Geometric Transformation/1
  Estimate Geometric Transformation/1 -> Apply Geometric Transformation/2
  Corner Locations/1(Pts) -> Data Type Conversion1/1
  "x, y, psi"/1 -> Selector3/1, Selector1/1
  Center Locations/2(Center) -> Corner Locations/2(Center)
  "Image "/1 -> Apply Geometric Transformation/1
  Apply Geometric Transformation/1 -> Image/1
  Unit Delay5/1 -> Angle from  horizontal axis/2
  Selector1/1 -> Difference/1
  Selector3/1 -> Difference1/1
  Difference/1 -> Angle from  horizontal axis/1
  Difference1/1 -> Gain/1
  Gain/1 -> Center Locations/1(Noise)

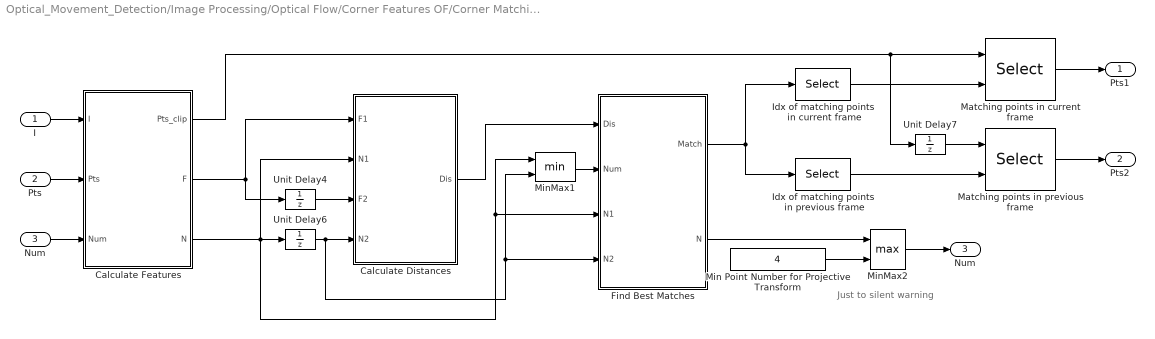
== system Optical_Movement_Detection/Image Processing/Optical Flow/Corner Features OF/Corner Matching ==
  note: Just to
      | silent warning
  I : Inport  OutDataType=sfix(16)  OutScaling=2^0
  Pts : Inport  Port=2  OutDataType=sfix(16)  OutScaling=2^0
  Num : Inport  Port=3  OutDataType=sfix(16)  OutScaling=2^0
  Calculate Distances : Subsystem  TreatAsAtomicUnit=on  mask{maxNum=maxNum}
      mask prompts: maxNum "Maximum data number:"
      settings: AttributesFormatString=between features.
  Calculate Features : Subsystem  TreatAsAtomicUnit=on  mask{winLen=winLen, maxNum=maxNum}
      mask prompts: winLen "Neighborhood size:"; maxNum "Maximum number of features:"
  Find Best Matches : Subsystem  TreatAsAtomicUnit=on  mask{maxNum=maxNum, threshold=threshold}
      mask prompts: maxNum "Maximum data number:"
      settings: AttributesFormatString=between the features\nin the current and previous frames
  Idx of matching points  in current frame : Selector  NumberOfDimensions=2  IndexMode=Zero-based  InputPortWidth=2  IndexOptions=Index vector (dialog),Select all  Indices=0,1  OutputSizes=1,1
  Idx of matching points  in previous frame : Selector  NumberOfDimensions=2  IndexMode=Zero-based  InputPortWidth=2  IndexOptions=Index vector (dialog),Select all  Indices=1,1  OutputSizes=1,1
  Matching points in current frame : Selector  NumberOfDimensions=2  IndexMode=Zero-based  InputPortWidth=2  IndexOptions=Select all,Index vector (port)  Indices=0,1  OutputSizes=1,1
  Matching points in previous frame : Selector  NumberOfDimensions=2  IndexMode=Zero-based  InputPortWidth=2  IndexOptions=Select all,Index vector (port)  Indices=0,1  OutputSizes=1,1
  Min Point Number for Projective Transform : Constant  Value=4  OutDataType=sfix(16)  OutScaling=2^0  OutDataTypeStr=Inherit: Inherit via back propagation
  MinMax1 : MinMax  Inputs=2  OutDataType=sfix(16)  OutScaling=2^0
  MinMax2 : MinMax  Function=max  Inputs=2  OutDataType=sfix(16)  OutScaling=2^0  OutDataTypeStr=Inherit: Inherit via back propagation
  Unit Delay4 : UnitDelay  SampleTime=-1
  Unit Delay6 : UnitDelay  SampleTime=-1
  Unit Delay7 : UnitDelay  SampleTime=-1
  Pts1 : Outport  OutDataType=sfix(16)  OutScaling=2^0
  Pts2 : Outport  Port=2  OutDataType=sfix(16)  OutScaling=2^0
  "Num " : Outport  Port=3  OutDataType=sfix(16)  OutScaling=2^0
  wires:
  Calculate Features/2(F) -> Calculate Distances/1(F1), Unit Delay4/1
  Calculate Features/3(N) -> Calculate Distances/2(N1), Unit Delay6/1, MinMax1/1, Find Best Matches/3(N1)
  Calculate Features/1(Pts_clip) -> Unit Delay7/1, Matching points in current frame/1
  Num/1 -> Calculate Features/3(Num)
  Unit Delay6/1 -> Calculate Distances/4(N2), MinMax1/2, Find Best Matches/4(N2)
  Unit Delay4/1 -> Calculate Distances/3(F2)
  Matching points in previous frame/1 -> Pts2/1
  Matching points in current frame/1 -> Pts1/1
  Unit Delay7/1 -> Matching points in previous frame/1
  Idx of matching points  in current frame/1 -> Matching points in current frame/2
  Idx of matching points  in previous frame/1 -> Matching points in previous frame/2
  Find Best Matches/1(Match) -> Idx of matching points  in previous frame/1, Idx of matching points  in current frame/1
  Calculate Distances/1(Dis) -> Find Best Matches/1(Dis)
  I/1 -> Calculate Features/1(I)
  Pts/1 -> Calculate Features/2(Pts)
  Min Point Number for Projective Transform/1 -> MinMax2/2
  Find Best Matches/2(N) -> MinMax2/1
  MinMax2/1 -> "Num "/1
  MinMax1/1 -> Find Best Matches/2(Num)

== system Optical_Movement_Detection/Image Processing/Input/Subsystem/Synthetic Video Generation1/Read Image ==
  Enable : EnablePort  PropagateVarSize=During execution
  Image From Workspace : vipsrcs/Image From Workspace  Tag=vipblks_nd  SystemSampleTime=-1  ImageValue=imresize(imread('concordaerial.png'), 0.5)  Ts=inf  imagePorts=One multidimensional signal  ImageDataType=single  Signed=on  WordLength=16  sdImageDataType=sfix(16)  FractionLengthMode=User-defined  FractionLength=15  OutPortLabels=R|G|B
  Probe : Probe  ProbeWidth=off  ProbeSampleTime=off  ProbeComplexSignal=off  ProbeSignalDimensions=on  ProbeDimensionsDataType=single
  Image : Outport  InitialOutput=0
  Size : Outport  Port=2
  wires:
  Image From Workspace/1 -> Probe/1, Image/1
  Probe/1 -> Size/1

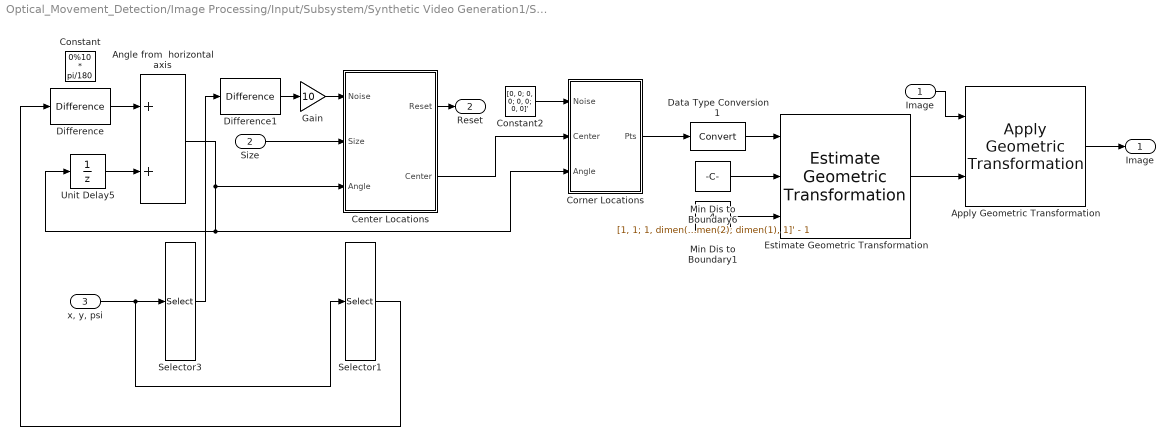
== system Optical_Movement_Detection/Image Processing/Input/Subsystem/Synthetic Video Generation1/Synthesize Video ==
  "Image " : Inport  OutDataType=sfix(16)  OutScaling=2^0
  Size : Inport  Port=2  OutDataType=sfix(16)  OutScaling=2^0
  "x, y, psi" : Inport  Port=3  OutDataType=sfix(16)  OutScaling=2^0
  Angle from  horizontal axis : Sum  OutDataType=sfix(16)  OutScaling=2^-10
  Apply Geometric Transformation : vipgeotforms/Apply Geometric Transformation  DialogController=vipDDGCreate  DialogControllerArgs=DataTag1  tformSource=Input port  tformValue=[1 0 0; 0 1 0; 0 0 1]  approxProjectiveFlag=off  errorTolerance=1.0  roiMethod=Whole input image  roiSource=Specify via dialog  roiBBox=[0 0 128 256]  roiVertice=[0 0 10 12 20 22]  inputClipFlag=off  interpolationMethod=Bilinear  fillValue=0  viewPortMethod=Specify via dialog  outputSize=dimen  outputLoc=[0 0]  outputClipFlag=off
  Center Locations : Subsystem
  Constant : Constant  Value=0%10 * pi/180  OutDataType=fixdt(1, 16)  OutScaling=2^0
  Constant2 : Constant  Value=[0, 0; 0, 0; 0, 0; 0, 0]'  OutDataType=fixdt(1, 16)  OutScaling=2^0
  Corner Locations : Subsystem
  Data Type Conversion1 : DataTypeConversion  OutDataType=sfix(16)  OutScaling=2^0
  Difference : simulink/Discrete/Difference  SystemSampleTime=-1  ICPrevInput=0.0  OutMin=[]  OutMax=[]  OutDataType=fixdt(1, 16)  OutScaling=2^-10  DoSatur=off
  Difference1 : simulink/Discrete/Difference  SystemSampleTime=-1  ICPrevInput=0.0  OutMin=[]  OutMax=[]  OutDataType=fixdt(1, 16)  OutScaling=2^-10  DoSatur=off
  Estimate Geometric Transformation : vipgeotforms/Estimate Geometric Transformation  DialogController=vipDDGCreate  DialogControllerArgs=DataTag3  tformType=Projective  isRandomSampling=off  algMethod=Random Sample Consensus (RANSAC)  numMethod=Specified value  isStopSampling=off  percentStop=75  distanceAlg=1.5  distanceGeo=1.5  sampleNum=100  maxSampleNum=200  desiredConfidence=99  isRefineTForm=off  isOutputInlier=off  outDT4IntInput=Obsolete10a  outDT4IntInputActive=Single  isVarSizeAllowed=off  isReleaseMode=on
  Gain : Gain  Gain=10  ParameterDataType=fixdt(1, 16)  ParameterScaling=2^0  OutDataType=fixdt(1, 16)  OutScaling=2^0
  Min Dis to Boundary1 : Constant  Value=4  OutDataType=sfix(16)  OutScaling=2^0  OutDataTypeStr=Inherit: Inherit via back propagation
  Min Dis to Boundary6 : Constant  Value=[1, 1; 1, dimen(2); dimen(1), dimen(2); dimen(1), 1]' - 1  OutDataType=sfix(16)  OutScaling=2^0  OutDataTypeStr=Inherit: Inherit via back propagation
  Selector1 : Selector  InputPortWidth=3  IndexOptions=Index vector (dialog)  Indices=[3]  OutputSizes=1
  Selector3 : Selector  InputPortWidth=3  IndexOptions=Index vector (dialog)  Indices=[1 2]  OutputSizes=1
  Unit Delay5 : UnitDelay  X0=-pi/12  SampleTime=-1
  Image : Outport  OutDataType=sfix(16)  OutScaling=2^0
  Reset : Outport  Port=2  OutDataType=sfix(16)  OutScaling=2^0
  wires:
  Constant2/1 -> Corner Locations/1(Noise)
  Angle from  horizontal axis/1 -> Center Locations/3(Angle), Corner Locations/3(Angle), Unit Delay5/1
  Center Locations/1(Reset) -> Reset/1
  Size/1 -> Center Locations/2(Size)
  Min Dis to Boundary6/1 -> Estimate Geometric Transformation/2
  Min Dis to Boundary1/1 -> Estimate Geometric Transformation/3
  Data Type Conversion1/1 -> Estimate Geometric Transformation/1
  Estimate Geometric Transformation/1 -> Apply Geometric Transformation/2
  Corner Locations/1(Pts) -> Data Type Conversion1/1
  "x, y, psi"/1 -> Selector3/1, Selector1/1
  Center Locations/2(Center) -> Corner Locations/2(Center)
  "Image "/1 -> Apply Geometric Transformation/1
  Apply Geometric Transformation/1 -> Image/1
  Unit Delay5/1 -> Angle from  horizontal axis/2
  Selector1/1 -> Difference/1
  Selector3/1 -> Difference1/1
  Difference/1 -> Angle from  horizontal axis/1
  Difference1/1 -> Gain/1
  Gain/1 -> Center Locations/1(Noise)
